simulink model "DoubleThermostat_diff"  (R2016b)
settings: Solver=VariableStepAuto  StartTime=0.0  StopTime=10.0  RelTol=1e-3
settings Model: Creator=live  LastModifiedBy=live

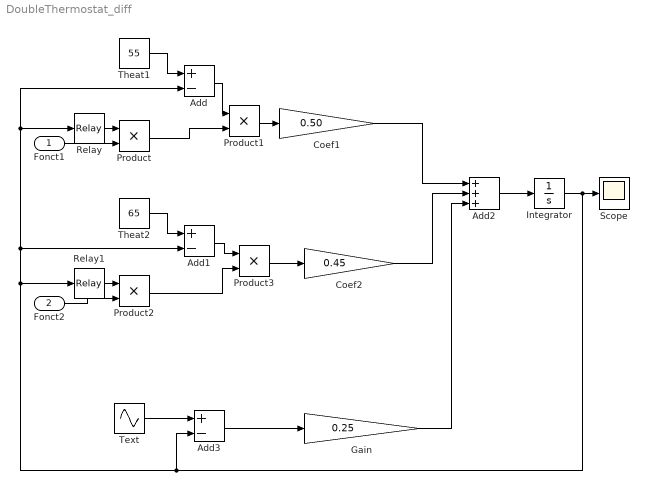
== system DoubleThermostat_diff ==
  Fonct1 : Inport
  Fonct2 : Inport  Port=2
  Add : Sum  Inputs=+-
  Add1 : Sum  Inputs=+-
  Add2 : Sum  Inputs=+++
  Add3 : Sum  Inputs=+-
  Coef1 : Gain  Gain=0.50
  Coef2 : Gain  Gain=0.45
  Gain : Gain  Gain=0.25
  Integrator : Integrator  InitialCondition=20
  Product{,1..3} (4 alike) : Product
  Relay : Relay  OnSwitchValue=24  OffSwitchValue=19  OnOutputValue=0  OffOutputValue=1
  Relay1 : Relay  OnSwitchValue=25  OffSwitchValue=20  OnOutputValue=0  OffOutputValue=1
  Scope : Scope
  Text : Sin  Amplitude=15  Bias=10  Frequency=0.04  SampleTime=0
  Theat1 : Constant  Value=55
  Theat2 : Constant  Value=65
  wires:
  Fonct1/1 -> Product/2
  Relay/1 -> Product/1
  Theat1/1 -> Add/1
  Integrator/1 -> Scope/1, Relay1/1, Add1/2, Add/2, Relay/1, Add3/2
  Product1/1 -> Coef1/1
  Add/1 -> Product1/1
  Product/1 -> Product1/2
  Relay1/1 -> Product2/1
  Fonct2/1 -> Product2/2
  Theat2/1 -> Add1/1
  Add1/1 -> Product3/1
  Product2/1 -> Product3/2
  Product3/1 -> Coef2/1
  Coef1/1 -> Add2/1
  Coef2/1 -> Add2/2
  Text/1 -> Add3/1
  Add3/1 -> Gain/1
  Gain/1 -> Add2/3
  Add2/1 -> Integrator/1
